simulink model "Calculator"  (R2024b)
settings: Solver=VariableStepAuto  StartTime=0.0  StopTime=10.0  RelTol=1e-3
(part 1 of 2)
settings Model: Creator=Ian  LastModifiedBy=Ian

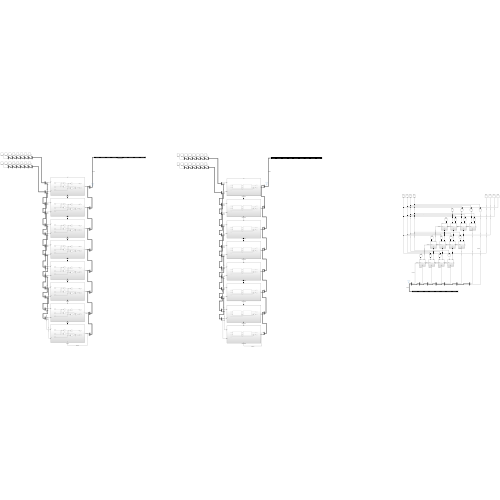
[thumbnail: Simulink's stored preview of the top-level diagram]
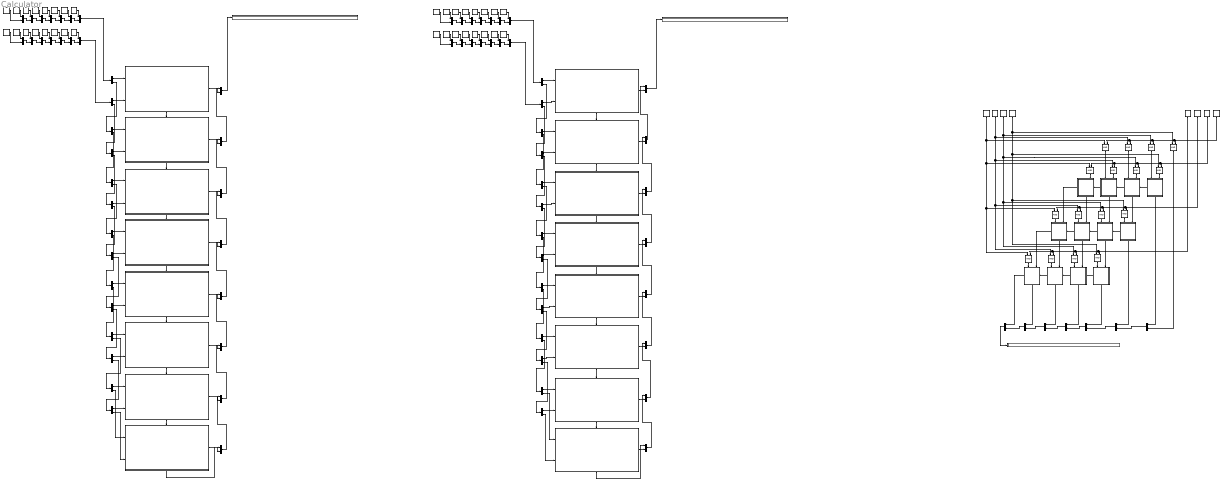
== system Calculator ==
  AND{,3..17} (16 alike) : Logic  IconShape=distinctive  AllPortsSameDT=off  OutDataTypeStr=boolean
  Add{11..13,15..18,21..25,27} (13 alike) : Constant  Value=0
  Add14 : Constant
  Add26 : Constant
  Add28 : Constant
  Adder : Subsystem
      settings: PortSchema="{\"entries\":[{\"content\":{\"sides\":[{\"content\":{\"connectorIds\":[\"In1\",\"In2\"]},\"type\":\"ConnectorPlacement.EquallySpacedRectSide\",\"uuid\":\"7bda4a13-5714-4766-b13e-fbedd8378c0d\"},{\"content\":{\"connectorIds\":[\"Out1\"],\"side\":\"RIGHT\"},\"type\":\"ConnectorPlacement.EquallySpacedRectSide\",\"uuid\":\"12590a9d-1e20-4d4b-a015-8cc67798c588\"},{\"content\":{\"connectorIds\":[\"In3\"],\"side\":\"TOP\"},\"type\":\"ConnectorPlacement.EquallySpacedRectSide\",\"uuid\":\"02eef574-06bf-4445-a216-f5494700e03c\"},{\"content\":{\"connectorIds\":[\"Out2\"],\"side\":\"BOTTOM\"},\"type\":\"ConnectorPlacement.EquallySpacedRectSide\",\"uuid\":\"95bb6c32-4776-4ae5-879f-000f498d11ec\"}]},\"type\":\"ConnectorPlacement.EquallySpacedConnector\",\"uuid\":\"b3982cbe-2d0c-455f-a3cf-748a4a59c66e\"}],\"packageUris\":[\"http://schema.mathworks.com/mf0/Connector/R2020b\"],\"version\":\"1.0\"}"
  Adder1 : Subsystem
      settings: PortSchema="{\"entries\":[{\"content\":{\"sides\":[{\"content\":{\"connectorIds\":[\"In1\",\"In2\"]},\"type\":\"ConnectorPlacement.EquallySpacedRectSide\",\"uuid\":\"7bda4a13-5714-4766-b13e-fbedd8378c0d\"},{\"content\":{\"connectorIds\":[\"Out1\"],\"side\":\"RIGHT\"},\"type\":\"ConnectorPlacement.EquallySpacedRectSide\",\"uuid\":\"12590a9d-1e20-4d4b-a015-8cc67798c588\"},{\"content\":{\"connectorIds\":[\"In3\"],\"side\":\"TOP\"},\"type\":\"ConnectorPlacement.EquallySpacedRectSide\",\"uuid\":\"02eef574-06bf-4445-a216-f5494700e03c\"},{\"content\":{\"connectorIds\":[\"Out2\"],\"side\":\"BOTTOM\"},\"type\":\"ConnectorPlacement.EquallySpacedRectSide\",\"uuid\":\"95bb6c32-4776-4ae5-879f-000f498d11ec\"}]},\"type\":\"ConnectorPlacement.EquallySpacedConnector\",\"uuid\":\"b3982cbe-2d0c-455f-a3cf-748a4a59c66e\"}],\"packageUris\":[\"http://schema.mathworks.com/mf0/Connector/R2020b\"],\"version\":\"1.0\"}"
  Adder10 : Subsystem
      settings: PortSchema="{\"entries\":[{\"content\":{\"sides\":[{\"content\":{\"connectorIds\":[\"In1\",\"In2\"]},\"type\":\"ConnectorPlacement.EquallySpacedRectSide\",\"uuid\":\"7bda4a13-5714-4766-b13e-fbedd8378c0d\"},{\"content\":{\"connectorIds\":[\"Out1\"],\"side\":\"RIGHT\"},\"type\":\"ConnectorPlacement.EquallySpacedRectSide\",\"uuid\":\"12590a9d-1e20-4d4b-a015-8cc67798c588\"},{\"content\":{\"connectorIds\":[\"In3\"],\"side\":\"TOP\"},\"type\":\"ConnectorPlacement.EquallySpacedRectSide\",\"uuid\":\"02eef574-06bf-4445-a216-f5494700e03c\"},{\"content\":{\"connectorIds\":[\"Out2\"],\"side\":\"BOTTOM\"},\"type\":\"ConnectorPlacement.EquallySpacedRectSide\",\"uuid\":\"95bb6c32-4776-4ae5-879f-000f498d11ec\"}]},\"type\":\"ConnectorPlacement.EquallySpacedConnector\",\"uuid\":\"b3982cbe-2d0c-455f-a3cf-748a4a59c66e\"}],\"packageUris\":[\"http://schema.mathworks.com/mf0/Connector/R2020b\"],\"version\":\"1.0\"}"
  Adder11 : Subsystem
      settings: PortSchema="{\"entries\":[{\"content\":{\"sides\":[{\"content\":{\"connectorIds\":[\"In1\",\"In2\"]},\"type\":\"ConnectorPlacement.EquallySpacedRectSide\",\"uuid\":\"7bda4a13-5714-4766-b13e-fbedd8378c0d\"},{\"content\":{\"connectorIds\":[\"Out1\"],\"side\":\"RIGHT\"},\"type\":\"ConnectorPlacement.EquallySpacedRectSide\",\"uuid\":\"12590a9d-1e20-4d4b-a015-8cc67798c588\"},{\"content\":{\"connectorIds\":[\"In3\"],\"side\":\"TOP\"},\"type\":\"ConnectorPlacement.EquallySpacedRectSide\",\"uuid\":\"02eef574-06bf-4445-a216-f5494700e03c\"},{\"content\":{\"connectorIds\":[\"Out2\"],\"side\":\"BOTTOM\"},\"type\":\"ConnectorPlacement.EquallySpacedRectSide\",\"uuid\":\"95bb6c32-4776-4ae5-879f-000f498d11ec\"}]},\"type\":\"ConnectorPlacement.EquallySpacedConnector\",\"uuid\":\"b3982cbe-2d0c-455f-a3cf-748a4a59c66e\"}],\"packageUris\":[\"http://schema.mathworks.com/mf0/Connector/R2020b\"],\"version\":\"1.0\"}"
  Adder12 : Subsystem
      settings: PortSchema="{\"entries\":[{\"content\":{\"sides\":[{\"content\":{\"connectorIds\":[\"In1\",\"In2\"]},\"type\":\"ConnectorPlacement.EquallySpacedRectSide\",\"uuid\":\"7bda4a13-5714-4766-b13e-fbedd8378c0d\"},{\"content\":{\"connectorIds\":[\"Out1\"],\"side\":\"RIGHT\"},\"type\":\"ConnectorPlacement.EquallySpacedRectSide\",\"uuid\":\"12590a9d-1e20-4d4b-a015-8cc67798c588\"},{\"content\":{\"connectorIds\":[\"In3\"],\"side\":\"TOP\"},\"type\":\"ConnectorPlacement.EquallySpacedRectSide\",\"uuid\":\"02eef574-06bf-4445-a216-f5494700e03c\"},{\"content\":{\"connectorIds\":[\"Out2\"],\"side\":\"BOTTOM\"},\"type\":\"ConnectorPlacement.EquallySpacedRectSide\",\"uuid\":\"95bb6c32-4776-4ae5-879f-000f498d11ec\"}]},\"type\":\"ConnectorPlacement.EquallySpacedConnector\",\"uuid\":\"b3982cbe-2d0c-455f-a3cf-748a4a59c66e\"}],\"packageUris\":[\"http://schema.mathworks.com/mf0/Connector/R2020b\"],\"version\":\"1.0\"}"
  Adder13 : Subsystem
      settings: PortSchema="{\"entries\":[{\"content\":{\"sides\":[{\"content\":{\"connectorIds\":[\"In1\",\"In2\"]},\"type\":\"ConnectorPlacement.EquallySpacedRectSide\",\"uuid\":\"7bda4a13-5714-4766-b13e-fbedd8378c0d\"},{\"content\":{\"connectorIds\":[\"Out1\"],\"side\":\"RIGHT\"},\"type\":\"ConnectorPlacement.EquallySpacedRectSide\",\"uuid\":\"12590a9d-1e20-4d4b-a015-8cc67798c588\"},{\"content\":{\"connectorIds\":[\"In3\"],\"side\":\"TOP\"},\"type\":\"ConnectorPlacement.EquallySpacedRectSide\",\"uuid\":\"02eef574-06bf-4445-a216-f5494700e03c\"},{\"content\":{\"connectorIds\":[\"Out2\"],\"side\":\"BOTTOM\"},\"type\":\"ConnectorPlacement.EquallySpacedRectSide\",\"uuid\":\"95bb6c32-4776-4ae5-879f-000f498d11ec\"}]},\"type\":\"ConnectorPlacement.EquallySpacedConnector\",\"uuid\":\"b3982cbe-2d0c-455f-a3cf-748a4a59c66e\"}],\"packageUris\":[\"http://schema.mathworks.com/mf0/Connector/R2020b\"],\"version\":\"1.0\"}"
  Adder14 : Subsystem
      settings: PortSchema="{\"entries\":[{\"content\":{\"sides\":[{\"content\":{\"connectorIds\":[\"In1\",\"In2\"]},\"type\":\"ConnectorPlacement.EquallySpacedRectSide\",\"uuid\":\"7bda4a13-5714-4766-b13e-fbedd8378c0d\"},{\"content\":{\"connectorIds\":[\"Out1\"],\"side\":\"RIGHT\"},\"type\":\"ConnectorPlacement.EquallySpacedRectSide\",\"uuid\":\"12590a9d-1e20-4d4b-a015-8cc67798c588\"},{\"content\":{\"connectorIds\":[\"In3\"],\"side\":\"TOP\"},\"type\":\"ConnectorPlacement.EquallySpacedRectSide\",\"uuid\":\"02eef574-06bf-4445-a216-f5494700e03c\"},{\"content\":{\"connectorIds\":[\"Out2\"],\"side\":\"BOTTOM\"},\"type\":\"ConnectorPlacement.EquallySpacedRectSide\",\"uuid\":\"95bb6c32-4776-4ae5-879f-000f498d11ec\"}]},\"type\":\"ConnectorPlacement.EquallySpacedConnector\",\"uuid\":\"b3982cbe-2d0c-455f-a3cf-748a4a59c66e\"}],\"packageUris\":[\"http://schema.mathworks.com/mf0/Connector/R2020b\"],\"version\":\"1.0\"}"
  Adder15 : Subsystem
      settings: PortSchema="{\"entries\":[{\"content\":{\"sides\":[{\"content\":{\"connectorIds\":[\"In1\",\"In2\"]},\"type\":\"ConnectorPlacement.EquallySpacedRectSide\",\"uuid\":\"7bda4a13-5714-4766-b13e-fbedd8378c0d\"},{\"content\":{\"connectorIds\":[\"Out1\"],\"side\":\"RIGHT\"},\"type\":\"ConnectorPlacement.EquallySpacedRectSide\",\"uuid\":\"12590a9d-1e20-4d4b-a015-8cc67798c588\"},{\"content\":{\"connectorIds\":[\"In3\"],\"side\":\"TOP\"},\"type\":\"ConnectorPlacement.EquallySpacedRectSide\",\"uuid\":\"02eef574-06bf-4445-a216-f5494700e03c\"},{\"content\":{\"connectorIds\":[\"Out2\"],\"side\":\"BOTTOM\"},\"type\":\"ConnectorPlacement.EquallySpacedRectSide\",\"uuid\":\"95bb6c32-4776-4ae5-879f-000f498d11ec\"}]},\"type\":\"ConnectorPlacement.EquallySpacedConnector\",\"uuid\":\"b3982cbe-2d0c-455f-a3cf-748a4a59c66e\"}],\"packageUris\":[\"http://schema.mathworks.com/mf0/Connector/R2020b\"],\"version\":\"1.0\"}"
  Adder16 : Subsystem
      settings: PortSchema="{\"entries\":[{\"content\":{\"sides\":[{\"content\":{\"connectorIds\":[\"In1\",\"In2\"]},\"type\":\"ConnectorPlacement.EquallySpacedRectSide\",\"uuid\":\"7bda4a13-5714-4766-b13e-fbedd8378c0d\"},{\"content\":{\"connectorIds\":[\"Out1\"],\"side\":\"RIGHT\"},\"type\":\"ConnectorPlacement.EquallySpacedRectSide\",\"uuid\":\"12590a9d-1e20-4d4b-a015-8cc67798c588\"},{\"content\":{\"connectorIds\":[\"In3\"],\"side\":\"TOP\"},\"type\":\"ConnectorPlacement.EquallySpacedRectSide\",\"uuid\":\"02eef574-06bf-4445-a216-f5494700e03c\"},{\"content\":{\"connectorIds\":[\"Out2\"],\"side\":\"BOTTOM\"},\"type\":\"ConnectorPlacement.EquallySpacedRectSide\",\"uuid\":\"95bb6c32-4776-4ae5-879f-000f498d11ec\"}]},\"type\":\"ConnectorPlacement.EquallySpacedConnector\",\"uuid\":\"b3982cbe-2d0c-455f-a3cf-748a4a59c66e\"}],\"packageUris\":[\"http://schema.mathworks.com/mf0/Connector/R2020b\"],\"version\":\"1.0\"}"
  Adder17 : Subsystem
      settings: PortSchema="{\"entries\":[{\"content\":{\"sides\":[{\"content\":{\"connectorIds\":[\"In1\",\"In2\"]},\"type\":\"ConnectorPlacement.EquallySpacedRectSide\",\"uuid\":\"7bda4a13-5714-4766-b13e-fbedd8378c0d\"},{\"content\":{\"connectorIds\":[\"Out1\"],\"side\":\"RIGHT\"},\"type\":\"ConnectorPlacement.EquallySpacedRectSide\",\"uuid\":\"12590a9d-1e20-4d4b-a015-8cc67798c588\"},{\"content\":{\"connectorIds\":[\"In3\"],\"side\":\"TOP\"},\"type\":\"ConnectorPlacement.EquallySpacedRectSide\",\"uuid\":\"02eef574-06bf-4445-a216-f5494700e03c\"},{\"content\":{\"connectorIds\":[\"Out2\"],\"side\":\"BOTTOM\"},\"type\":\"ConnectorPlacement.EquallySpacedRectSide\",\"uuid\":\"95bb6c32-4776-4ae5-879f-000f498d11ec\"}]},\"type\":\"ConnectorPlacement.EquallySpacedConnector\",\"uuid\":\"b3982cbe-2d0c-455f-a3cf-748a4a59c66e\"}],\"packageUris\":[\"http://schema.mathworks.com/mf0/Connector/R2020b\"],\"version\":\"1.0\"}"
  Adder18 : Subsystem
      settings: PortSchema="{\"entries\":[{\"content\":{\"sides\":[{\"content\":{\"connectorIds\":[\"In1\",\"In2\"]},\"type\":\"ConnectorPlacement.EquallySpacedRectSide\",\"uuid\":\"7bda4a13-5714-4766-b13e-fbedd8378c0d\"},{\"content\":{\"connectorIds\":[\"Out1\"],\"side\":\"RIGHT\"},\"type\":\"ConnectorPlacement.EquallySpacedRectSide\",\"uuid\":\"12590a9d-1e20-4d4b-a015-8cc67798c588\"},{\"content\":{\"connectorIds\":[\"In3\"],\"side\":\"TOP\"},\"type\":\"ConnectorPlacement.EquallySpacedRectSide\",\"uuid\":\"02eef574-06bf-4445-a216-f5494700e03c\"},{\"content\":{\"connectorIds\":[\"Out2\"],\"side\":\"BOTTOM\"},\"type\":\"ConnectorPlacement.EquallySpacedRectSide\",\"uuid\":\"95bb6c32-4776-4ae5-879f-000f498d11ec\"}]},\"type\":\"ConnectorPlacement.EquallySpacedConnector\",\"uuid\":\"b3982cbe-2d0c-455f-a3cf-748a4a59c66e\"}],\"packageUris\":[\"http://schema.mathworks.com/mf0/Connector/R2020b\"],\"version\":\"1.0\"}"
  Adder19 : Subsystem
      settings: PortSchema="{\"entries\":[{\"content\":{\"sides\":[{\"content\":{\"connectorIds\":[\"In1\",\"In2\"]},\"type\":\"ConnectorPlacement.EquallySpacedRectSide\",\"uuid\":\"7bda4a13-5714-4766-b13e-fbedd8378c0d\"},{\"content\":{\"connectorIds\":[\"Out1\"],\"side\":\"RIGHT\"},\"type\":\"ConnectorPlacement.EquallySpacedRectSide\",\"uuid\":\"12590a9d-1e20-4d4b-a015-8cc67798c588\"},{\"content\":{\"connectorIds\":[\"In3\"],\"side\":\"TOP\"},\"type\":\"ConnectorPlacement.EquallySpacedRectSide\",\"uuid\":\"02eef574-06bf-4445-a216-f5494700e03c\"},{\"content\":{\"connectorIds\":[\"Out2\"],\"side\":\"BOTTOM\"},\"type\":\"ConnectorPlacement.EquallySpacedRectSide\",\"uuid\":\"95bb6c32-4776-4ae5-879f-000f498d11ec\"}]},\"type\":\"ConnectorPlacement.EquallySpacedConnector\",\"uuid\":\"b3982cbe-2d0c-455f-a3cf-748a4a59c66e\"}],\"packageUris\":[\"http://schema.mathworks.com/mf0/Connector/R2020b\"],\"version\":\"1.0\"}"
  Adder2 : Subsystem
      settings: PortSchema="{\"entries\":[{\"content\":{\"sides\":[{\"content\":{\"connectorIds\":[\"In1\",\"In2\"]},\"type\":\"ConnectorPlacement.EquallySpacedRectSide\",\"uuid\":\"7bda4a13-5714-4766-b13e-fbedd8378c0d\"},{\"content\":{\"connectorIds\":[\"Out1\"],\"side\":\"RIGHT\"},\"type\":\"ConnectorPlacement.EquallySpacedRectSide\",\"uuid\":\"12590a9d-1e20-4d4b-a015-8cc67798c588\"},{\"content\":{\"connectorIds\":[\"In3\"],\"side\":\"TOP\"},\"type\":\"ConnectorPlacement.EquallySpacedRectSide\",\"uuid\":\"02eef574-06bf-4445-a216-f5494700e03c\"},{\"content\":{\"connectorIds\":[\"Out2\"],\"side\":\"BOTTOM\"},\"type\":\"ConnectorPlacement.EquallySpacedRectSide\",\"uuid\":\"95bb6c32-4776-4ae5-879f-000f498d11ec\"}]},\"type\":\"ConnectorPlacement.EquallySpacedConnector\",\"uuid\":\"b3982cbe-2d0c-455f-a3cf-748a4a59c66e\"}],\"packageUris\":[\"http://schema.mathworks.com/mf0/Connector/R2020b\"],\"version\":\"1.0\"}"
  Adder3 : Subsystem
      settings: PortSchema="{\"entries\":[{\"content\":{\"sides\":[{\"content\":{\"connectorIds\":[\"In1\",\"In2\"]},\"type\":\"ConnectorPlacement.EquallySpacedRectSide\",\"uuid\":\"7bda4a13-5714-4766-b13e-fbedd8378c0d\"},{\"content\":{\"connectorIds\":[\"Out1\"],\"side\":\"RIGHT\"},\"type\":\"ConnectorPlacement.EquallySpacedRectSide\",\"uuid\":\"12590a9d-1e20-4d4b-a015-8cc67798c588\"},{\"content\":{\"connectorIds\":[\"In3\"],\"side\":\"TOP\"},\"type\":\"ConnectorPlacement.EquallySpacedRectSide\",\"uuid\":\"02eef574-06bf-4445-a216-f5494700e03c\"},{\"content\":{\"connectorIds\":[\"Out2\"],\"side\":\"BOTTOM\"},\"type\":\"ConnectorPlacement.EquallySpacedRectSide\",\"uuid\":\"95bb6c32-4776-4ae5-879f-000f498d11ec\"}]},\"type\":\"ConnectorPlacement.EquallySpacedConnector\",\"uuid\":\"b3982cbe-2d0c-455f-a3cf-748a4a59c66e\"}],\"packageUris\":[\"http://schema.mathworks.com/mf0/Connector/R2020b\"],\"version\":\"1.0\"}"
  Adder4 : Subsystem
      settings: PortSchema="{\"entries\":[{\"content\":{\"sides\":[{\"content\":{\"connectorIds\":[\"In1\",\"In2\"]},\"type\":\"ConnectorPlacement.EquallySpacedRectSide\",\"uuid\":\"7bda4a13-5714-4766-b13e-fbedd8378c0d\"},{\"content\":{\"connectorIds\":[\"Out1\"],\"side\":\"RIGHT\"},\"type\":\"ConnectorPlacement.EquallySpacedRectSide\",\"uuid\":\"12590a9d-1e20-4d4b-a015-8cc67798c588\"},{\"content\":{\"connectorIds\":[\"In3\"],\"side\":\"TOP\"},\"type\":\"ConnectorPlacement.EquallySpacedRectSide\",\"uuid\":\"02eef574-06bf-4445-a216-f5494700e03c\"},{\"content\":{\"connectorIds\":[\"Out2\"],\"side\":\"BOTTOM\"},\"type\":\"ConnectorPlacement.EquallySpacedRectSide\",\"uuid\":\"95bb6c32-4776-4ae5-879f-000f498d11ec\"}]},\"type\":\"ConnectorPlacement.EquallySpacedConnector\",\"uuid\":\"b3982cbe-2d0c-455f-a3cf-748a4a59c66e\"}],\"packageUris\":[\"http://schema.mathworks.com/mf0/Connector/R2020b\"],\"version\":\"1.0\"}"
  Adder5 : Subsystem
      settings: PortSchema="{\"entries\":[{\"content\":{\"sides\":[{\"content\":{\"connectorIds\":[\"In1\",\"In2\"]},\"type\":\"ConnectorPlacement.EquallySpacedRectSide\",\"uuid\":\"7bda4a13-5714-4766-b13e-fbedd8378c0d\"},{\"content\":{\"connectorIds\":[\"Out1\"],\"side\":\"RIGHT\"},\"type\":\"ConnectorPlacement.EquallySpacedRectSide\",\"uuid\":\"12590a9d-1e20-4d4b-a015-8cc67798c588\"},{\"content\":{\"connectorIds\":[\"In3\"],\"side\":\"TOP\"},\"type\":\"ConnectorPlacement.EquallySpacedRectSide\",\"uuid\":\"02eef574-06bf-4445-a216-f5494700e03c\"},{\"content\":{\"connectorIds\":[\"Out2\"],\"side\":\"BOTTOM\"},\"type\":\"ConnectorPlacement.EquallySpacedRectSide\",\"uuid\":\"95bb6c32-4776-4ae5-879f-000f498d11ec\"}]},\"type\":\"ConnectorPlacement.EquallySpacedConnector\",\"uuid\":\"b3982cbe-2d0c-455f-a3cf-748a4a59c66e\"}],\"packageUris\":[\"http://schema.mathworks.com/mf0/Connector/R2020b\"],\"version\":\"1.0\"}"
  Adder6 : Subsystem
      settings: PortSchema="{\"entries\":[{\"content\":{\"sides\":[{\"content\":{\"connectorIds\":[\"In1\",\"In2\"]},\"type\":\"ConnectorPlacement.EquallySpacedRectSide\",\"uuid\":\"7bda4a13-5714-4766-b13e-fbedd8378c0d\"},{\"content\":{\"connectorIds\":[\"Out1\"],\"side\":\"RIGHT\"},\"type\":\"ConnectorPlacement.EquallySpacedRectSide\",\"uuid\":\"12590a9d-1e20-4d4b-a015-8cc67798c588\"},{\"content\":{\"connectorIds\":[\"In3\"],\"side\":\"TOP\"},\"type\":\"ConnectorPlacement.EquallySpacedRectSide\",\"uuid\":\"02eef574-06bf-4445-a216-f5494700e03c\"},{\"content\":{\"connectorIds\":[\"Out2\"],\"side\":\"BOTTOM\"},\"type\":\"ConnectorPlacement.EquallySpacedRectSide\",\"uuid\":\"95bb6c32-4776-4ae5-879f-000f498d11ec\"}]},\"type\":\"ConnectorPlacement.EquallySpacedConnector\",\"uuid\":\"b3982cbe-2d0c-455f-a3cf-748a4a59c66e\"}],\"packageUris\":[\"http://schema.mathworks.com/mf0/Connector/R2020b\"],\"version\":\"1.0\"}"
  Adder7 : Subsystem
      settings: PortSchema="{\"entries\":[{\"content\":{\"sides\":[{\"content\":{\"connectorIds\":[\"In1\",\"In2\"]},\"type\":\"ConnectorPlacement.EquallySpacedRectSide\",\"uuid\":\"7bda4a13-5714-4766-b13e-fbedd8378c0d\"},{\"content\":{\"connectorIds\":[\"Out1\"],\"side\":\"RIGHT\"},\"type\":\"ConnectorPlacement.EquallySpacedRectSide\",\"uuid\":\"12590a9d-1e20-4d4b-a015-8cc67798c588\"},{\"content\":{\"connectorIds\":[\"In3\"],\"side\":\"TOP\"},\"type\":\"ConnectorPlacement.EquallySpacedRectSide\",\"uuid\":\"02eef574-06bf-4445-a216-f5494700e03c\"},{\"content\":{\"connectorIds\":[\"Out2\"],\"side\":\"BOTTOM\"},\"type\":\"ConnectorPlacement.EquallySpacedRectSide\",\"uuid\":\"95bb6c32-4776-4ae5-879f-000f498d11ec\"}]},\"type\":\"ConnectorPlacement.EquallySpacedConnector\",\"uuid\":\"b3982cbe-2d0c-455f-a3cf-748a4a59c66e\"}],\"packageUris\":[\"http://schema.mathworks.com/mf0/Connector/R2020b\"],\"version\":\"1.0\"}"
  Adder8 : Subsystem
      settings: PortSchema="{\"entries\":[{\"content\":{\"sides\":[{\"content\":{\"connectorIds\":[\"In1\",\"In2\"]},\"type\":\"ConnectorPlacement.EquallySpacedRectSide\",\"uuid\":\"7bda4a13-5714-4766-b13e-fbedd8378c0d\"},{\"content\":{\"connectorIds\":[\"Out1\"],\"side\":\"RIGHT\"},\"type\":\"ConnectorPlacement.EquallySpacedRectSide\",\"uuid\":\"12590a9d-1e20-4d4b-a015-8cc67798c588\"},{\"content\":{\"connectorIds\":[\"In3\"],\"side\":\"TOP\"},\"type\":\"ConnectorPlacement.EquallySpacedRectSide\",\"uuid\":\"02eef574-06bf-4445-a216-f5494700e03c\"},{\"content\":{\"connectorIds\":[\"Out2\"],\"side\":\"BOTTOM\"},\"type\":\"ConnectorPlacement.EquallySpacedRectSide\",\"uuid\":\"95bb6c32-4776-4ae5-879f-000f498d11ec\"}]},\"type\":\"ConnectorPlacement.EquallySpacedConnector\",\"uuid\":\"b3982cbe-2d0c-455f-a3cf-748a4a59c66e\"}],\"packageUris\":[\"http://schema.mathworks.com/mf0/Connector/R2020b\"],\"version\":\"1.0\"}"
  Adder9 : Subsystem
      settings: PortSchema="{\"entries\":[{\"content\":{\"sides\":[{\"content\":{\"connectorIds\":[\"In1\",\"In2\"]},\"type\":\"ConnectorPlacement.EquallySpacedRectSide\",\"uuid\":\"7bda4a13-5714-4766-b13e-fbedd8378c0d\"},{\"content\":{\"connectorIds\":[\"Out1\"],\"side\":\"RIGHT\"},\"type\":\"ConnectorPlacement.EquallySpacedRectSide\",\"uuid\":\"12590a9d-1e20-4d4b-a015-8cc67798c588\"},{\"content\":{\"connectorIds\":[\"In3\"],\"side\":\"TOP\"},\"type\":\"ConnectorPlacement.EquallySpacedRectSide\",\"uuid\":\"02eef574-06bf-4445-a216-f5494700e03c\"},{\"content\":{\"connectorIds\":[\"Out2\"],\"side\":\"BOTTOM\"},\"type\":\"ConnectorPlacement.EquallySpacedRectSide\",\"uuid\":\"95bb6c32-4776-4ae5-879f-000f498d11ec\"}]},\"type\":\"ConnectorPlacement.EquallySpacedConnector\",\"uuid\":\"b3982cbe-2d0c-455f-a3cf-748a4a59c66e\"}],\"packageUris\":[\"http://schema.mathworks.com/mf0/Connector/R2020b\"],\"version\":\"1.0\"}"
  AdditionDisplay : Display
  Bus Creator{,1..50} (51 alike) : BusCreator  Inputs=2
  Bus Selector{,1..27} (28 alike) : BusSelector  OutputSignals=signal1,signal2
  Display : Display
  Display1 : Display
  Mult{11..14,24} (5 alike) : Constant
  Mult21 : Constant  Value=0
  Mult22 : Constant  Value=0
  Mult23 : Constant  Value=0
  Sub{11..14,16,18,21..24,26,28} (12 alike) : Constant  Value=0
  Sub{15,17,25,27} (4 alike) : Constant
  Subtractor1 : Subsystem
      settings: PortSchema="{\"entries\":[{\"content\":{\"sides\":[{\"content\":{\"connectorIds\":[\"In1\",\"In2\"]},\"type\":\"ConnectorPlacement.EquallySpacedRectSide\",\"uuid\":\"7bda4a13-5714-4766-b13e-fbedd8378c0d\"},{\"content\":{\"connectorIds\":[\"Out1\"],\"side\":\"RIGHT\"},\"type\":\"ConnectorPlacement.EquallySpacedRectSide\",\"uuid\":\"12590a9d-1e20-4d4b-a015-8cc67798c588\"},{\"content\":{\"connectorIds\":[\"In3\"],\"side\":\"TOP\"},\"type\":\"ConnectorPlacement.EquallySpacedRectSide\",\"uuid\":\"02eef574-06bf-4445-a216-f5494700e03c\"},{\"content\":{\"connectorIds\":[\"Out2\"],\"side\":\"BOTTOM\"},\"type\":\"ConnectorPlacement.EquallySpacedRectSide\",\"uuid\":\"e8f31c1b-a942-47d5-ae1c-1de8906fe25d\"}]},\"type\":\"ConnectorPlacement.EquallySpacedConnector\",\"uuid\":\"b3982cbe-2d0c-455f-a3cf-748a4a59c66e\"}],\"packageUris\":[\"http://schema.mathworks.com/mf0/Connector/R2020b\"],\"version\":\"1.0\"}"
  Subtractor2 : Subsystem
      settings: PortSchema="{\"entries\":[{\"content\":{\"sides\":[{\"content\":{\"connectorIds\":[\"In1\",\"In2\"]},\"type\":\"ConnectorPlacement.EquallySpacedRectSide\",\"uuid\":\"7bda4a13-5714-4766-b13e-fbedd8378c0d\"},{\"content\":{\"connectorIds\":[\"Out1\"],\"side\":\"RIGHT\"},\"type\":\"ConnectorPlacement.EquallySpacedRectSide\",\"uuid\":\"12590a9d-1e20-4d4b-a015-8cc67798c588\"},{\"content\":{\"connectorIds\":[\"In3\"],\"side\":\"TOP\"},\"type\":\"ConnectorPlacement.EquallySpacedRectSide\",\"uuid\":\"02eef574-06bf-4445-a216-f5494700e03c\"},{\"content\":{\"connectorIds\":[\"Out2\"],\"side\":\"BOTTOM\"},\"type\":\"ConnectorPlacement.EquallySpacedRectSide\",\"uuid\":\"e8f31c1b-a942-47d5-ae1c-1de8906fe25d\"}]},\"type\":\"ConnectorPlacement.EquallySpacedConnector\",\"uuid\":\"b3982cbe-2d0c-455f-a3cf-748a4a59c66e\"}],\"packageUris\":[\"http://schema.mathworks.com/mf0/Connector/R2020b\"],\"version\":\"1.0\"}"
  Subtractor3 : Subsystem
      settings: PortSchema="{\"entries\":[{\"content\":{\"sides\":[{\"content\":{\"connectorIds\":[\"In1\",\"In2\"]},\"type\":\"ConnectorPlacement.EquallySpacedRectSide\",\"uuid\":\"7bda4a13-5714-4766-b13e-fbedd8378c0d\"},{\"content\":{\"connectorIds\":[\"Out1\"],\"side\":\"RIGHT\"},\"type\":\"ConnectorPlacement.EquallySpacedRectSide\",\"uuid\":\"12590a9d-1e20-4d4b-a015-8cc67798c588\"},{\"content\":{\"connectorIds\":[\"In3\"],\"side\":\"TOP\"},\"type\":\"ConnectorPlacement.EquallySpacedRectSide\",\"uuid\":\"02eef574-06bf-4445-a216-f5494700e03c\"},{\"content\":{\"connectorIds\":[\"Out2\"],\"side\":\"BOTTOM\"},\"type\":\"ConnectorPlacement.EquallySpacedRectSide\",\"uuid\":\"e8f31c1b-a942-47d5-ae1c-1de8906fe25d\"}]},\"type\":\"ConnectorPlacement.EquallySpacedConnector\",\"uuid\":\"b3982cbe-2d0c-455f-a3cf-748a4a59c66e\"}],\"packageUris\":[\"http://schema.mathworks.com/mf0/Connector/R2020b\"],\"version\":\"1.0\"}"
  Subtractor4 : Subsystem
      settings: PortSchema="{\"entries\":[{\"content\":{\"sides\":[{\"content\":{\"connectorIds\":[\"In1\",\"In2\"]},\"type\":\"ConnectorPlacement.EquallySpacedRectSide\",\"uuid\":\"7bda4a13-5714-4766-b13e-fbedd8378c0d\"},{\"content\":{\"connectorIds\":[\"Out1\"],\"side\":\"RIGHT\"},\"type\":\"ConnectorPlacement.EquallySpacedRectSide\",\"uuid\":\"12590a9d-1e20-4d4b-a015-8cc67798c588\"},{\"content\":{\"connectorIds\":[\"In3\"],\"side\":\"TOP\"},\"type\":\"ConnectorPlacement.EquallySpacedRectSide\",\"uuid\":\"02eef574-06bf-4445-a216-f5494700e03c\"},{\"content\":{\"connectorIds\":[\"Out2\"],\"side\":\"BOTTOM\"},\"type\":\"ConnectorPlacement.EquallySpacedRectSide\",\"uuid\":\"e8f31c1b-a942-47d5-ae1c-1de8906fe25d\"}]},\"type\":\"ConnectorPlacement.EquallySpacedConnector\",\"uuid\":\"b3982cbe-2d0c-455f-a3cf-748a4a59c66e\"}],\"packageUris\":[\"http://schema.mathworks.com/mf0/Connector/R2020b\"],\"version\":\"1.0\"}"
  Subtractor5 : Subsystem
      settings: PortSchema="{\"entries\":[{\"content\":{\"sides\":[{\"content\":{\"connectorIds\":[\"In1\",\"In2\"]},\"type\":\"ConnectorPlacement.EquallySpacedRectSide\",\"uuid\":\"7bda4a13-5714-4766-b13e-fbedd8378c0d\"},{\"content\":{\"connectorIds\":[\"Out1\"],\"side\":\"RIGHT\"},\"type\":\"ConnectorPlacement.EquallySpacedRectSide\",\"uuid\":\"12590a9d-1e20-4d4b-a015-8cc67798c588\"},{\"content\":{\"connectorIds\":[\"In3\"],\"side\":\"TOP\"},\"type\":\"ConnectorPlacement.EquallySpacedRectSide\",\"uuid\":\"02eef574-06bf-4445-a216-f5494700e03c\"},{\"content\":{\"connectorIds\":[\"Out2\"],\"side\":\"BOTTOM\"},\"type\":\"ConnectorPlacement.EquallySpacedRectSide\",\"uuid\":\"e8f31c1b-a942-47d5-ae1c-1de8906fe25d\"}]},\"type\":\"ConnectorPlacement.EquallySpacedConnector\",\"uuid\":\"b3982cbe-2d0c-455f-a3cf-748a4a59c66e\"}],\"packageUris\":[\"http://schema.mathworks.com/mf0/Connector/R2020b\"],\"version\":\"1.0\"}"
  Subtractor6 : Subsystem
      settings: PortSchema="{\"entries\":[{\"content\":{\"sides\":[{\"content\":{\"connectorIds\":[\"In1\",\"In2\"]},\"type\":\"ConnectorPlacement.EquallySpacedRectSide\",\"uuid\":\"7bda4a13-5714-4766-b13e-fbedd8378c0d\"},{\"content\":{\"connectorIds\":[\"Out1\"],\"side\":\"RIGHT\"},\"type\":\"ConnectorPlacement.EquallySpacedRectSide\",\"uuid\":\"12590a9d-1e20-4d4b-a015-8cc67798c588\"},{\"content\":{\"connectorIds\":[\"In3\"],\"side\":\"TOP\"},\"type\":\"ConnectorPlacement.EquallySpacedRectSide\",\"uuid\":\"02eef574-06bf-4445-a216-f5494700e03c\"},{\"content\":{\"connectorIds\":[\"Out2\"],\"side\":\"BOTTOM\"},\"type\":\"ConnectorPlacement.EquallySpacedRectSide\",\"uuid\":\"e8f31c1b-a942-47d5-ae1c-1de8906fe25d\"}]},\"type\":\"ConnectorPlacement.EquallySpacedConnector\",\"uuid\":\"b3982cbe-2d0c-455f-a3cf-748a4a59c66e\"}],\"packageUris\":[\"http://schema.mathworks.com/mf0/Connector/R2020b\"],\"version\":\"1.0\"}"
  Subtractor7 : Subsystem
      settings: PortSchema="{\"entries\":[{\"content\":{\"sides\":[{\"content\":{\"connectorIds\":[\"In1\",\"In2\"]},\"type\":\"ConnectorPlacement.EquallySpacedRectSide\",\"uuid\":\"7bda4a13-5714-4766-b13e-fbedd8378c0d\"},{\"content\":{\"connectorIds\":[\"Out1\"],\"side\":\"RIGHT\"},\"type\":\"ConnectorPlacement.EquallySpacedRectSide\",\"uuid\":\"12590a9d-1e20-4d4b-a015-8cc67798c588\"},{\"content\":{\"connectorIds\":[\"In3\"],\"side\":\"TOP\"},\"type\":\"ConnectorPlacement.EquallySpacedRectSide\",\"uuid\":\"02eef574-06bf-4445-a216-f5494700e03c\"},{\"content\":{\"connectorIds\":[\"Out2\"],\"side\":\"BOTTOM\"},\"type\":\"ConnectorPlacement.EquallySpacedRectSide\",\"uuid\":\"e8f31c1b-a942-47d5-ae1c-1de8906fe25d\"}]},\"type\":\"ConnectorPlacement.EquallySpacedConnector\",\"uuid\":\"b3982cbe-2d0c-455f-a3cf-748a4a59c66e\"}],\"packageUris\":[\"http://schema.mathworks.com/mf0/Connector/R2020b\"],\"version\":\"1.0\"}"
  Subtractor8 : Subsystem
      settings: PortSchema="{\"entries\":[{\"content\":{\"sides\":[{\"content\":{\"connectorIds\":[\"In1\",\"In2\"]},\"type\":\"ConnectorPlacement.EquallySpacedRectSide\",\"uuid\":\"7bda4a13-5714-4766-b13e-fbedd8378c0d\"},{\"content\":{\"connectorIds\":[\"Out1\"],\"side\":\"RIGHT\"},\"type\":\"ConnectorPlacement.EquallySpacedRectSide\",\"uuid\":\"12590a9d-1e20-4d4b-a015-8cc67798c588\"},{\"content\":{\"connectorIds\":[\"In3\"],\"side\":\"TOP\"},\"type\":\"ConnectorPlacement.EquallySpacedRectSide\",\"uuid\":\"02eef574-06bf-4445-a216-f5494700e03c\"},{\"content\":{\"connectorIds\":[\"Out2\"],\"side\":\"BOTTOM\"},\"type\":\"ConnectorPlacement.EquallySpacedRectSide\",\"uuid\":\"e8f31c1b-a942-47d5-ae1c-1de8906fe25d\"}]},\"type\":\"ConnectorPlacement.EquallySpacedConnector\",\"uuid\":\"b3982cbe-2d0c-455f-a3cf-748a4a59c66e\"}],\"packageUris\":[\"http://schema.mathworks.com/mf0/Connector/R2020b\"],\"version\":\"1.0\"}"
  wires:
  Adder/2(Out2) -> Adder1/3(In3)
  Adder1/2(Out2) -> Adder2/3(In3)
  Adder2/2(Out2) -> Adder3/3(In3)
  Adder5/2(Out2) -> Adder6/3(In3)
  Adder6/2(Out2) -> Adder7/3(In3)
  Adder4/2(Out2) -> Adder5/3(In3)
  Adder3/2(Out2) -> Adder4/3(In3)
  Add12/1 -> Bus Creator8/1
  Add11/1 -> Bus Creator8/2
  Add13/1 -> Bus Creator9/1
  Bus Creator8/1 -> Bus Creator9/2
  Add15/1 -> Bus Creator11/1
  Add14/1 -> Bus Creator10/1
  Bus Creator9/1 -> Bus Creator10/2
  Bus Creator10/1 -> Bus Creator11/2
  Add16/1 -> Bus Creator14/1
  Add17/1 -> Bus Creator12/1
  Add18/1 -> Bus Creator13/1
  Bus Creator11/1 -> Bus Creator14/2
  Bus Creator14/1 -> Bus Creator12/2
  Bus Creator12/1 -> Bus Creator13/2
  Bus Creator19/1 -> Bus Creator17/2
  Bus Creator17/1 -> Bus Creator18/2
  Add23/1 -> Bus Creator21/1
  Add28/1 -> Bus Creator18/1
  Bus Creator20/1 -> Bus Creator21/2
  Bus Creator16/1 -> Bus Creator19/2
  Add25/1 -> Bus Creator16/1
  Add27/1 -> Bus Creator17/1
  Bus Creator21/1 -> Bus Creator15/2
  Add24/1 -> Bus Creator15/1
  Add22/1 -> Bus Creator20/1
  Add21/1 -> Bus Creator20/2
  Bus Creator15/1 -> Bus Creator16/2
  Add26/1 -> Bus Creator19/1
  Bus Selector/1 -> Adder/1(In1)  "<signal1>"
  Bus Selector/2 -> Bus Selector1/1  "<signal2>"
  Bus Selector2/1 -> Adder/2(In2)  "<signal1>"
  Bus Selector2/2 -> Bus Selector3/1  "<signal2>"
  Bus Selector1/1 -> Adder1/1(In1)  "<signal1>"
  Bus Selector3/1 -> Adder1/2(In2)  "<signal1>"
  Bus Selector6/2 -> Bus Selector7/1  "<signal2>"
  Bus Selector5/1 -> Adder3/1(In1)  "<signal1>"
  Bus Selector7/1 -> Adder3/2(In2)  "<signal1>"
  Bus Selector4/1 -> Adder2/1(In1)  "<signal1>"
  Bus Selector4/2 -> Bus Selector5/1  "<signal2>"
  Bus Selector6/1 -> Adder2/2(In2)  "<signal1>"
  Bus Selector3/2 -> Bus Selector6/1  "<signal2>"
  Bus Selector1/2 -> Bus Selector4/1  "<signal2>"
  Bus Selector8/2 -> Bus Selector10/1  "<signal2>"
  Bus Selector9/2 -> Bus Selector12/1  "<signal2>"
  Bus Selector10/2 -> Bus Selector11/1  "<signal2>"
  Bus Selector12/2 -> Bus Selector13/1  "<signal2>"
  Bus Selector5/2 -> Bus Selector8/1  "<signal2>"
  Bus Selector7/2 -> Bus Selector9/1  "<signal2>"
  Bus Selector8/1 -> Adder4/1(In1)  "<signal1>"
  Bus Selector9/1 -> Adder4/2(In2)  "<signal1>"
  Bus Selector13/1 -> Adder6/2(In2)  "<signal1>"
  Bus Selector11/1 -> Adder6/1(In1)  "<signal1>"
  Bus Selector12/1 -> Adder5/2(In2)  "<signal1>"
  Bus Selector10/1 -> Adder5/1(In1)  "<signal1>"
  Bus Creator18/1 -> Bus Selector2/1
  Bus Creator13/1 -> Bus Selector/1
  Bus Selector11/2 -> Adder7/1(In1)  "<signal2>"
  Bus Selector13/2 -> Adder7/2(In2)  "<signal2>"
  Adder7/2(Out2) -> Bus Creator/1  "AddOut9"
  Adder7/1(Out1) -> Bus Creator/2  "AddOut8"
  Bus Creator/1 -> Bus Creator1/1
  Adder6/1(Out1) -> Bus Creator1/2  "AddOut7"
  Bus Creator1/1 -> Bus Creator2/1
  Adder5/1(Out1) -> Bus Creator2/2  "AddOut6"
  Bus Creator2/1 -> Bus Creator3/1
  Adder4/1(Out1) -> Bus Creator3/2  "AddOut5"
  Bus Creator3/1 -> Bus Creator4/1
  Adder3/1(Out1) -> Bus Creator4/2  "AddOut4"
  Adder2/1(Out1) -> Bus Creator5/2  "AddOut3"
  Bus Creator4/1 -> Bus Creator5/1
  Bus Creator5/1 -> Bus Creator6/1
  Adder1/1(Out1) -> Bus Creator6/2  "AddOut2"
  Bus Creator6/1 -> Bus Creator7/1
  Adder/1(Out1) -> Bus Creator7/2  "AddOut1"
  Bus Creator7/1 -> AdditionDisplay/1  "AddBus"
  Subtractor1/1(Out1) -> Bus Creator41/2  "SubOut1"
  Subtractor6/1(Out1) -> Bus Creator34/2  "SubOut6"
  Subtractor8/1(Out1) -> Bus Creator22/2  "SubOut8"
  Subtractor8/2(Out2) -> Bus Creator22/1  "SubOut9"
  Subtractor3/1(Out1) -> Bus Creator39/2  "SubOut3"
  Subtractor4/1(Out1) -> Bus Creator38/2  "SubOut4"
  Bus Selector20/2 -> Bus Selector21/1  "<signal2>"
  Bus Creator27/1 -> Bus Selector14/1
  Bus Selector15/1 -> Subtractor2/1(In1)  "<signal1>"
  Bus Selector27/1 -> Subtractor5/2(In2)  "<signal1>"
  Bus Selector15/2 -> Bus Selector22/1  "<signal2>"
  Bus Selector17/2 -> Subtractor8/1(In1)  "<signal2>"
  Bus Selector21/1 -> Subtractor2/2(In2)  "<signal1>"
  Bus Selector23/1 -> Subtractor4/1(In1)  "<signal1>"
  Bus Selector22/1 -> Subtractor3/1(In1)  "<signal1>"
  Bus Selector25/2 -> Bus Selector27/1  "<signal2>"
  Sub22/1 -> Bus Creator35/1
  Sub25/1 -> Bus Creator30/1
  Bus Creator30/1 -> Bus Creator33/2
  Bus Creator33/1 -> Bus Creator31/2
  Bus Selector14/2 -> Bus Selector15/1  "<signal2>"
  Bus Selector16/1 -> Subtractor6/1(In1)  "<signal1>"
  Bus Creator28/1 -> Bus Creator26/2
  Bus Creator40/1 -> Bus Creator41/1
  Bus Creator22/1 -> Bus Creator23/1
  Sub13/1 -> Bus Creator43/1
  Bus Creator32/1 -> Bus Selector20/1
  Sub18/1 -> Bus Creator27/1
  Bus Selector26/1 -> Subtractor5/1(In1)  "<signal1>"
  Bus Creator42/1 -> Bus Creator43/2
  Bus Creator25/1 -> Bus Creator28/2
  Sub28/1 -> Bus Creator32/1
  Bus Selector23/2 -> Bus Selector26/1  "<signal2>"
  Bus Selector18/2 -> Bus Selector19/1  "<signal2>"
  Sub23/1 -> Bus Creator36/1
  Bus Selector27/2 -> Bus Selector18/1  "<signal2>"
  Subtractor2/1(Out1) -> Bus Creator40/2  "SubOut2"
  Bus Creator39/1 -> Bus Creator40/1
  Bus Selector26/2 -> Bus Selector16/1  "<signal2>"
  Bus Selector14/1 -> Subtractor1/1(In1)  "<signal1>"
  Bus Creator29/1 -> Bus Creator30/2
  Bus Selector20/1 -> Subtractor1/2(In2)  "<signal1>"
  Bus Selector16/2 -> Bus Selector17/1  "<signal2>"
  Sub11/1 -> Bus Creator42/2
  Bus Creator23/1 -> Bus Creator34/1
  Sub12/1 -> Bus Creator42/1
  Bus Selector24/1 -> Subtractor3/2(In2)  "<signal1>"
  Sub24/1 -> Bus Creator29/1
  Bus Creator26/1 -> Bus Creator27/2
  Sub26/1 -> Bus Creator33/1
  Bus Selector19/1 -> Subtractor7/2(In2)  "<signal1>"
  Sub14/1 -> Bus Creator24/1
  Bus Creator41/1 -> Display1/1  "SubBus"
  Sub15/1 -> Bus Creator25/1
  Subtractor4/2(Out2) -> Subtractor5/3(In3)
  Bus Creator31/1 -> Bus Creator32/2
  Sub21/1 -> Bus Creator35/2
  Bus Selector22/2 -> Bus Selector23/1  "<signal2>"
  Bus Selector24/2 -> Bus Selector25/1  "<signal2>"
  Subtractor5/1(Out1) -> Bus Creator37/2  "SubOut5"
  Bus Creator43/1 -> Bus Creator24/2
  Bus Creator37/1 -> Bus Creator38/1
  Bus Selector21/2 -> Bus Selector24/1  "<signal2>"
  Bus Creator38/1 -> Bus Creator39/1
  Sub27/1 -> Bus Creator31/1
  Sub17/1 -> Bus Creator26/1
  Bus Creator35/1 -> Bus Creator36/2
  Bus Creator24/1 -> Bus Creator25/2
  Sub16/1 -> Bus Creator28/1
  Bus Creator36/1 -> Bus Creator29/2
  Bus Creator34/1 -> Bus Creator37/1
  Bus Selector17/1 -> Subtractor7/1(In1)  "<signal1>"
  Subtractor1/2(Out2) -> Subtractor2/3(In3)
  Subtractor2/2(Out2) -> Subtractor3/3(In3)
  Subtractor3/2(Out2) -> Subtractor4/3(In3)
  Bus Selector25/1 -> Subtractor4/2(In2)  "<signal1>"
  Bus Selector18/1 -> Subtractor6/2(In2)  "<signal1>"
  Subtractor6/2(Out2) -> Subtractor7/3(In3)
  Subtractor7/2(Out2) -> Subtractor8/3(In3)
  Subtractor7/1(Out1) -> Bus Creator23/2  "SubOut7"
  Bus Selector19/2 -> Subtractor8/2(In2)  "<signal2>"
  Subtractor5/2(Out2) -> Subtractor6/3(In3)
  Adder10/2(Carry) -> Adder11/3(In3)
  Adder9/2(Carry) -> Adder10/3(In3)
  Adder8/2(Carry) -> Adder9/3(In3)
  Mult24/1 -> AND8/2, AND6/2, AND4/2, AND/2
  Mult23/1 -> AND9/2, AND7/2, AND5/2, AND3/2
  Adder11/2(Carry) -> Adder13/1(In1)
  AND13/1 -> Adder13/2(In2)
  AND10/1 -> Adder14/2(In2)
  Adder14/2(Carry) -> Adder15/3(In3)
  Adder9/1(Out) -> Adder14/1(In1)
  AND12/1 -> Adder12/2(In2)
  Adder11/1(Out) -> Adder12/1(In1)
  Adder10/1(Out) -> Adder15/1(In1)
  AND11/1 -> Adder15/2(In2)
  Adder15/2(Carry) -> Adder12/3(In3)
  Mult22/1 -> AND13/2, AND12/2, AND11/2, AND10/2
  Adder12/2(Carry) -> Adder13/3(In3)
  AND3/1 -> Adder8/1(In1)
  AND4/1 -> Adder8/2(In2)
  AND5/1 -> Adder9/1(In1)
  AND6/1 -> Adder9/2(In2)
  AND8/1 -> Adder10/2(In2)
  AND9/1 -> Adder11/1(In1)
  AND/1 -> Bus Creator44/2  "MultOut8"
  Adder8/1(Out) -> Bus Creator44/1  "MultOut7"
  Adder13/1(Out) -> Adder16/1(In1)
  Adder15/1(Out) -> Adder18/1(In1)
  Mult13/1 -> AND4/1, AND5/1, AND15/1, AND11/1
  Adder12/1(Out) -> Adder19/1(In1)
  Mult11/1 -> AND8/1, AND9/1, AND13/1, AND17/1
  Mult12/1 -> AND6/1, AND7/1, AND16/1, AND12/1
  Adder16/2(Carry) -> Adder17/3(In3)
  AND14/1 -> Adder18/2(In2)
  Adder18/2(Carry) -> Adder19/3(In3)
  AND17/1 -> Adder17/2(In2)
  Mult21/1 -> AND17/2, AND16/2, AND15/2, AND14/2
  AND16/1 -> Adder16/2(In2)
  Adder13/2(Carry) -> Adder17/1(In1)
  AND15/1 -> Adder19/2(In2)
  Mult14/1 -> AND/1, AND3/1, AND14/1, AND10/1
  Adder19/2(Carry) -> Adder16/3(In3)
  Adder14/1(Out) -> Bus Creator45/1  "MultOut6"
  Adder18/1(Out) -> Bus Creator46/1  "MultOut5"
  Adder19/1(Out) -> Bus Creator47/1  "MultOut4"
  Adder16/1(Out) -> Bus Creator48/1  "MultOut3"
  Adder17/1(Out) -> Bus Creator49/1  "MultOut2"
  Adder17/2(Carry) -> Bus Creator50/1  "MultOut1"
  AND7/1 -> Adder10/1(In1)
  Bus Creator44/1 -> Bus Creator45/2
  Bus Creator45/1 -> Bus Creator46/2
  Bus Creator46/1 -> Bus Creator47/2
  Bus Creator47/1 -> Bus Creator48/2
  Bus Creator48/1 -> Bus Creator49/2
  Bus Creator49/1 -> Bus Creator50/2
  Bus Creator50/1 -> Display/1  "MultBus"

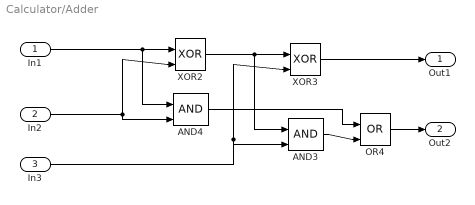
== system Calculator/Adder ==
  In1 : Inport
  In2 : Inport  Port=2
  In3 : Inport  Port=3
  AND3 : Logic  IconShape=distinctive  AllPortsSameDT=off  OutDataTypeStr=boolean
  AND4 : Logic  IconShape=distinctive  AllPortsSameDT=off  OutDataTypeStr=boolean
  OR4 : Logic  Operator=OR  IconShape=distinctive  AllPortsSameDT=off  OutDataTypeStr=boolean
  XOR2 : Logic  Operator=XOR  IconShape=distinctive  AllPortsSameDT=off  OutDataTypeStr=boolean
  XOR3 : Logic  Operator=XOR  IconShape=distinctive  AllPortsSameDT=off  OutDataTypeStr=boolean
  Out1 : Outport
  Out2 : Outport  Port=2
  wires:
  In2/1 -> AND4/2, XOR2/2
  AND3/1 -> OR4/2
  In3/1 -> XOR3/2, AND3/2
  In1/1 -> AND4/1, XOR2/1
  XOR3/1 -> Out1/1
  OR4/1 -> Out2/1
  AND4/1 -> OR4/1
  XOR2/1 -> AND3/1, XOR3/1

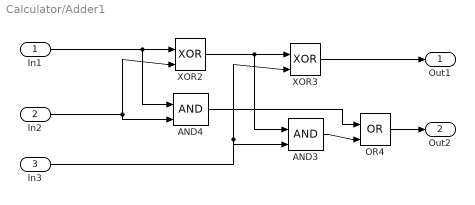
== system Calculator/Adder1 ==
  In1 : Inport
  In2 : Inport  Port=2
  In3 : Inport  Port=3
  AND3 : Logic  IconShape=distinctive  AllPortsSameDT=off  OutDataTypeStr=boolean
  AND4 : Logic  IconShape=distinctive  AllPortsSameDT=off  OutDataTypeStr=boolean
  OR4 : Logic  Operator=OR  IconShape=distinctive  AllPortsSameDT=off  OutDataTypeStr=boolean
  XOR2 : Logic  Operator=XOR  IconShape=distinctive  AllPortsSameDT=off  OutDataTypeStr=boolean
  XOR3 : Logic  Operator=XOR  IconShape=distinctive  AllPortsSameDT=off  OutDataTypeStr=boolean
  Out1 : Outport
  Out2 : Outport  Port=2
  wires:
  In2/1 -> AND4/2, XOR2/2
  AND3/1 -> OR4/2
  In3/1 -> XOR3/2, AND3/2
  In1/1 -> AND4/1, XOR2/1
  XOR3/1 -> Out1/1
  OR4/1 -> Out2/1
  AND4/1 -> OR4/1
  XOR2/1 -> AND3/1, XOR3/1

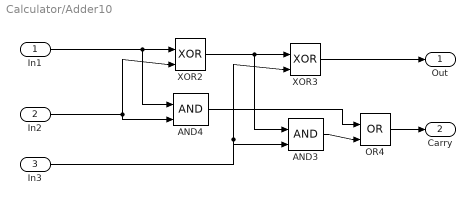
== system Calculator/Adder10 ==
  In1 : Inport
  In2 : Inport  Port=2
  In3 : Inport  Port=3
  AND3 : Logic  IconShape=distinctive  AllPortsSameDT=off  OutDataTypeStr=boolean
  AND4 : Logic  IconShape=distinctive  AllPortsSameDT=off  OutDataTypeStr=boolean
  OR4 : Logic  Operator=OR  IconShape=distinctive  AllPortsSameDT=off  OutDataTypeStr=boolean
  XOR2 : Logic  Operator=XOR  IconShape=distinctive  AllPortsSameDT=off  OutDataTypeStr=boolean
  XOR3 : Logic  Operator=XOR  IconShape=distinctive  AllPortsSameDT=off  OutDataTypeStr=boolean
  Out : Outport
  Carry : Outport  Port=2
  wires:
  In2/1 -> AND4/2, XOR2/2
  AND3/1 -> OR4/2
  In3/1 -> XOR3/2, AND3/2
  In1/1 -> AND4/1, XOR2/1
  XOR3/1 -> Out/1
  OR4/1 -> Carry/1
  AND4/1 -> OR4/1
  XOR2/1 -> AND3/1, XOR3/1

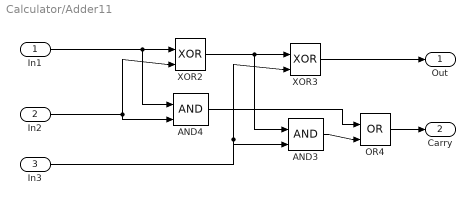
== system Calculator/Adder11 ==
  In1 : Inport
  In2 : Inport  Port=2
  In3 : Inport  Port=3
  AND3 : Logic  IconShape=distinctive  AllPortsSameDT=off  OutDataTypeStr=boolean
  AND4 : Logic  IconShape=distinctive  AllPortsSameDT=off  OutDataTypeStr=boolean
  OR4 : Logic  Operator=OR  IconShape=distinctive  AllPortsSameDT=off  OutDataTypeStr=boolean
  XOR2 : Logic  Operator=XOR  IconShape=distinctive  AllPortsSameDT=off  OutDataTypeStr=boolean
  XOR3 : Logic  Operator=XOR  IconShape=distinctive  AllPortsSameDT=off  OutDataTypeStr=boolean
  Out : Outport
  Carry : Outport  Port=2
  wires:
  In2/1 -> AND4/2, XOR2/2
  AND3/1 -> OR4/2
  In3/1 -> XOR3/2, AND3/2
  In1/1 -> AND4/1, XOR2/1
  XOR3/1 -> Out/1
  OR4/1 -> Carry/1
  AND4/1 -> OR4/1
  XOR2/1 -> AND3/1, XOR3/1

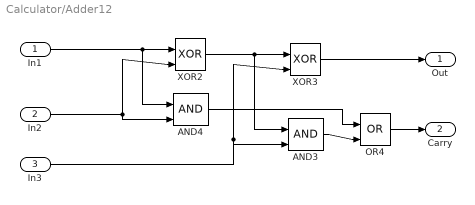
== system Calculator/Adder12 ==
  In1 : Inport
  In2 : Inport  Port=2
  In3 : Inport  Port=3
  AND3 : Logic  IconShape=distinctive  AllPortsSameDT=off  OutDataTypeStr=boolean
  AND4 : Logic  IconShape=distinctive  AllPortsSameDT=off  OutDataTypeStr=boolean
  OR4 : Logic  Operator=OR  IconShape=distinctive  AllPortsSameDT=off  OutDataTypeStr=boolean
  XOR2 : Logic  Operator=XOR  IconShape=distinctive  AllPortsSameDT=off  OutDataTypeStr=boolean
  XOR3 : Logic  Operator=XOR  IconShape=distinctive  AllPortsSameDT=off  OutDataTypeStr=boolean
  Out : Outport
  Carry : Outport  Port=2
  wires:
  In2/1 -> AND4/2, XOR2/2
  AND3/1 -> OR4/2
  In3/1 -> XOR3/2, AND3/2
  In1/1 -> AND4/1, XOR2/1
  XOR3/1 -> Out/1
  OR4/1 -> Carry/1
  AND4/1 -> OR4/1
  XOR2/1 -> AND3/1, XOR3/1

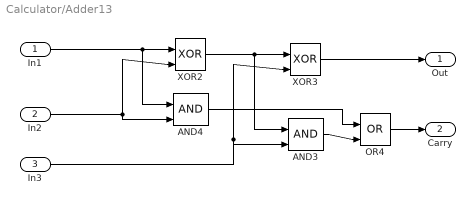
== system Calculator/Adder13 ==
  In1 : Inport
  In2 : Inport  Port=2
  In3 : Inport  Port=3
  AND3 : Logic  IconShape=distinctive  AllPortsSameDT=off  OutDataTypeStr=boolean
  AND4 : Logic  IconShape=distinctive  AllPortsSameDT=off  OutDataTypeStr=boolean
  OR4 : Logic  Operator=OR  IconShape=distinctive  AllPortsSameDT=off  OutDataTypeStr=boolean
  XOR2 : Logic  Operator=XOR  IconShape=distinctive  AllPortsSameDT=off  OutDataTypeStr=boolean
  XOR3 : Logic  Operator=XOR  IconShape=distinctive  AllPortsSameDT=off  OutDataTypeStr=boolean
  Out : Outport
  Carry : Outport  Port=2
  wires:
  In2/1 -> AND4/2, XOR2/2
  AND3/1 -> OR4/2
  In3/1 -> XOR3/2, AND3/2
  In1/1 -> AND4/1, XOR2/1
  XOR3/1 -> Out/1
  OR4/1 -> Carry/1
  AND4/1 -> OR4/1
  XOR2/1 -> AND3/1, XOR3/1

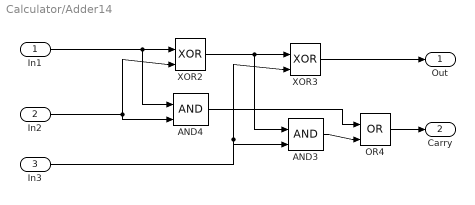
== system Calculator/Adder14 ==
  In1 : Inport
  In2 : Inport  Port=2
  In3 : Inport  Port=3
  AND3 : Logic  IconShape=distinctive  AllPortsSameDT=off  OutDataTypeStr=boolean
  AND4 : Logic  IconShape=distinctive  AllPortsSameDT=off  OutDataTypeStr=boolean
  OR4 : Logic  Operator=OR  IconShape=distinctive  AllPortsSameDT=off  OutDataTypeStr=boolean
  XOR2 : Logic  Operator=XOR  IconShape=distinctive  AllPortsSameDT=off  OutDataTypeStr=boolean
  XOR3 : Logic  Operator=XOR  IconShape=distinctive  AllPortsSameDT=off  OutDataTypeStr=boolean
  Out : Outport
  Carry : Outport  Port=2
  wires:
  In2/1 -> AND4/2, XOR2/2
  AND3/1 -> OR4/2
  In3/1 -> XOR3/2, AND3/2
  In1/1 -> AND4/1, XOR2/1
  XOR3/1 -> Out/1
  OR4/1 -> Carry/1
  AND4/1 -> OR4/1
  XOR2/1 -> AND3/1, XOR3/1

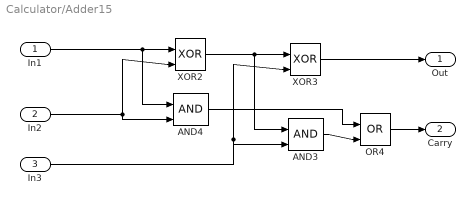
== system Calculator/Adder15 ==
  In1 : Inport
  In2 : Inport  Port=2
  In3 : Inport  Port=3
  AND3 : Logic  IconShape=distinctive  AllPortsSameDT=off  OutDataTypeStr=boolean
  AND4 : Logic  IconShape=distinctive  AllPortsSameDT=off  OutDataTypeStr=boolean
  OR4 : Logic  Operator=OR  IconShape=distinctive  AllPortsSameDT=off  OutDataTypeStr=boolean
  XOR2 : Logic  Operator=XOR  IconShape=distinctive  AllPortsSameDT=off  OutDataTypeStr=boolean
  XOR3 : Logic  Operator=XOR  IconShape=distinctive  AllPortsSameDT=off  OutDataTypeStr=boolean
  Out : Outport
  Carry : Outport  Port=2
  wires:
  In2/1 -> AND4/2, XOR2/2
  AND3/1 -> OR4/2
  In3/1 -> XOR3/2, AND3/2
  In1/1 -> AND4/1, XOR2/1
  XOR3/1 -> Out/1
  OR4/1 -> Carry/1
  AND4/1 -> OR4/1
  XOR2/1 -> AND3/1, XOR3/1

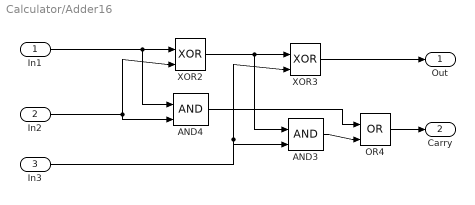
== system Calculator/Adder16 ==
  In1 : Inport
  In2 : Inport  Port=2
  In3 : Inport  Port=3
  AND3 : Logic  IconShape=distinctive  AllPortsSameDT=off  OutDataTypeStr=boolean
  AND4 : Logic  IconShape=distinctive  AllPortsSameDT=off  OutDataTypeStr=boolean
  OR4 : Logic  Operator=OR  IconShape=distinctive  AllPortsSameDT=off  OutDataTypeStr=boolean
  XOR2 : Logic  Operator=XOR  IconShape=distinctive  AllPortsSameDT=off  OutDataTypeStr=boolean
  XOR3 : Logic  Operator=XOR  IconShape=distinctive  AllPortsSameDT=off  OutDataTypeStr=boolean
  Out : Outport
  Carry : Outport  Port=2
  wires:
  In2/1 -> AND4/2, XOR2/2
  AND3/1 -> OR4/2
  In3/1 -> XOR3/2, AND3/2
  In1/1 -> AND4/1, XOR2/1
  XOR3/1 -> Out/1
  OR4/1 -> Carry/1
  AND4/1 -> OR4/1
  XOR2/1 -> AND3/1, XOR3/1

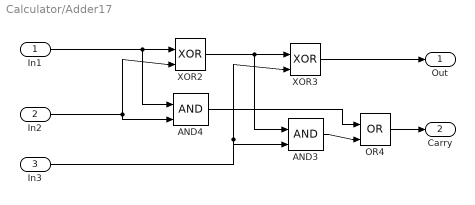
== system Calculator/Adder17 ==
  In1 : Inport
  In2 : Inport  Port=2
  In3 : Inport  Port=3
  AND3 : Logic  IconShape=distinctive  AllPortsSameDT=off  OutDataTypeStr=boolean
  AND4 : Logic  IconShape=distinctive  AllPortsSameDT=off  OutDataTypeStr=boolean
  OR4 : Logic  Operator=OR  IconShape=distinctive  AllPortsSameDT=off  OutDataTypeStr=boolean
  XOR2 : Logic  Operator=XOR  IconShape=distinctive  AllPortsSameDT=off  OutDataTypeStr=boolean
  XOR3 : Logic  Operator=XOR  IconShape=distinctive  AllPortsSameDT=off  OutDataTypeStr=boolean
  Out : Outport
  Carry : Outport  Port=2
  wires:
  In2/1 -> AND4/2, XOR2/2
  AND3/1 -> OR4/2
  In3/1 -> XOR3/2, AND3/2
  In1/1 -> AND4/1, XOR2/1
  XOR3/1 -> Out/1
  OR4/1 -> Carry/1
  AND4/1 -> OR4/1
  XOR2/1 -> AND3/1, XOR3/1

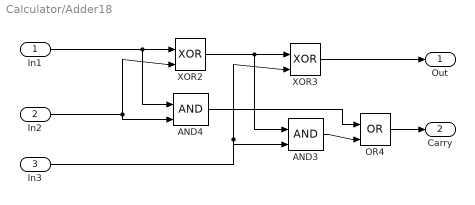
== system Calculator/Adder18 ==
  In1 : Inport
  In2 : Inport  Port=2
  In3 : Inport  Port=3
  AND3 : Logic  IconShape=distinctive  AllPortsSameDT=off  OutDataTypeStr=boolean
  AND4 : Logic  IconShape=distinctive  AllPortsSameDT=off  OutDataTypeStr=boolean
  OR4 : Logic  Operator=OR  IconShape=distinctive  AllPortsSameDT=off  OutDataTypeStr=boolean
  XOR2 : Logic  Operator=XOR  IconShape=distinctive  AllPortsSameDT=off  OutDataTypeStr=boolean
  XOR3 : Logic  Operator=XOR  IconShape=distinctive  AllPortsSameDT=off  OutDataTypeStr=boolean
  Out : Outport
  Carry : Outport  Port=2
  wires:
  In2/1 -> AND4/2, XOR2/2
  AND3/1 -> OR4/2
  In3/1 -> XOR3/2, AND3/2
  In1/1 -> AND4/1, XOR2/1
  XOR3/1 -> Out/1
  OR4/1 -> Carry/1
  AND4/1 -> OR4/1
  XOR2/1 -> AND3/1, XOR3/1

== system Calculator/Adder19 ==
  In1 : Inport
  In2 : Inport  Port=2
  In3 : Inport  Port=3
  AND3 : Logic  IconShape=distinctive  AllPortsSameDT=off  OutDataTypeStr=boolean
  AND4 : Logic  IconShape=distinctive  AllPortsSameDT=off  OutDataTypeStr=boolean
  OR4 : Logic  Operator=OR  IconShape=distinctive  AllPortsSameDT=off  OutDataTypeStr=boolean
  XOR2 : Logic  Operator=XOR  IconShape=distinctive  AllPortsSameDT=off  OutDataTypeStr=boolean
  XOR3 : Logic  Operator=XOR  IconShape=distinctive  AllPortsSameDT=off  OutDataTypeStr=boolean
  Out : Outport
  Carry : Outport  Port=2
  wires:
  In2/1 -> AND4/2, XOR2/2
  AND3/1 -> OR4/2
  In3/1 -> XOR3/2, AND3/2
  In1/1 -> AND4/1, XOR2/1
  XOR3/1 -> Out/1
  OR4/1 -> Carry/1
  AND4/1 -> OR4/1
  XOR2/1 -> AND3/1, XOR3/1

== system Calculator/Adder2 ==
  In1 : Inport
  In2 : Inport  Port=2
  In3 : Inport  Port=3
  AND3 : Logic  IconShape=distinctive  AllPortsSameDT=off  OutDataTypeStr=boolean
  AND4 : Logic  IconShape=distinctive  AllPortsSameDT=off  OutDataTypeStr=boolean
  OR4 : Logic  Operator=OR  IconShape=distinctive  AllPortsSameDT=off  OutDataTypeStr=boolean
  XOR2 : Logic  Operator=XOR  IconShape=distinctive  AllPortsSameDT=off  OutDataTypeStr=boolean
  XOR3 : Logic  Operator=XOR  IconShape=distinctive  AllPortsSameDT=off  OutDataTypeStr=boolean
  Out1 : Outport
  Out2 : Outport  Port=2
  wires:
  In2/1 -> AND4/2, XOR2/2
  AND3/1 -> OR4/2
  In3/1 -> XOR3/2, AND3/2
  In1/1 -> AND4/1, XOR2/1
  XOR3/1 -> Out1/1
  OR4/1 -> Out2/1
  AND4/1 -> OR4/1
  XOR2/1 -> AND3/1, XOR3/1

== system Calculator/Adder3 ==
  In1 : Inport
  In2 : Inport  Port=2
  In3 : Inport  Port=3
  AND3 : Logic  IconShape=distinctive  AllPortsSameDT=off  OutDataTypeStr=boolean
  AND4 : Logic  IconShape=distinctive  AllPortsSameDT=off  OutDataTypeStr=boolean
  OR4 : Logic  Operator=OR  IconShape=distinctive  AllPortsSameDT=off  OutDataTypeStr=boolean
  XOR2 : Logic  Operator=XOR  IconShape=distinctive  AllPortsSameDT=off  OutDataTypeStr=boolean
  XOR3 : Logic  Operator=XOR  IconShape=distinctive  AllPortsSameDT=off  OutDataTypeStr=boolean
  Out1 : Outport
  Out2 : Outport  Port=2
  wires:
  In2/1 -> AND4/2, XOR2/2
  AND3/1 -> OR4/2
  In3/1 -> XOR3/2, AND3/2
  In1/1 -> AND4/1, XOR2/1
  XOR3/1 -> Out1/1
  OR4/1 -> Out2/1
  AND4/1 -> OR4/1
  XOR2/1 -> AND3/1, XOR3/1

== system Calculator/Adder4 ==
  In1 : Inport
  In2 : Inport  Port=2
  In3 : Inport  Port=3
  AND3 : Logic  IconShape=distinctive  AllPortsSameDT=off  OutDataTypeStr=boolean
  AND4 : Logic  IconShape=distinctive  AllPortsSameDT=off  OutDataTypeStr=boolean
  OR4 : Logic  Operator=OR  IconShape=distinctive  AllPortsSameDT=off  OutDataTypeStr=boolean
  XOR2 : Logic  Operator=XOR  IconShape=distinctive  AllPortsSameDT=off  OutDataTypeStr=boolean
  XOR3 : Logic  Operator=XOR  IconShape=distinctive  AllPortsSameDT=off  OutDataTypeStr=boolean
  Out1 : Outport
  Out2 : Outport  Port=2
  wires:
  In2/1 -> AND4/2, XOR2/2
  AND3/1 -> OR4/2
  In3/1 -> XOR3/2, AND3/2
  In1/1 -> AND4/1, XOR2/1
  XOR3/1 -> Out1/1
  OR4/1 -> Out2/1
  AND4/1 -> OR4/1
  XOR2/1 -> AND3/1, XOR3/1

== system Calculator/Adder5 ==
  In1 : Inport
  In2 : Inport  Port=2
  In3 : Inport  Port=3
  AND3 : Logic  IconShape=distinctive  AllPortsSameDT=off  OutDataTypeStr=boolean
  AND4 : Logic  IconShape=distinctive  AllPortsSameDT=off  OutDataTypeStr=boolean
  OR4 : Logic  Operator=OR  IconShape=distinctive  AllPortsSameDT=off  OutDataTypeStr=boolean
  XOR2 : Logic  Operator=XOR  IconShape=distinctive  AllPortsSameDT=off  OutDataTypeStr=boolean
  XOR3 : Logic  Operator=XOR  IconShape=distinctive  AllPortsSameDT=off  OutDataTypeStr=boolean
  Out1 : Outport
  Out2 : Outport  Port=2
  wires:
  In2/1 -> AND4/2, XOR2/2
  AND3/1 -> OR4/2
  In3/1 -> XOR3/2, AND3/2
  In1/1 -> AND4/1, XOR2/1
  XOR3/1 -> Out1/1
  OR4/1 -> Out2/1
  AND4/1 -> OR4/1
  XOR2/1 -> AND3/1, XOR3/1

== system Calculator/Adder6 ==
  In1 : Inport
  In2 : Inport  Port=2
  In3 : Inport  Port=3
  AND3 : Logic  IconShape=distinctive  AllPortsSameDT=off  OutDataTypeStr=boolean
  AND4 : Logic  IconShape=distinctive  AllPortsSameDT=off  OutDataTypeStr=boolean
  OR4 : Logic  Operator=OR  IconShape=distinctive  AllPortsSameDT=off  OutDataTypeStr=boolean
  XOR2 : Logic  Operator=XOR  IconShape=distinctive  AllPortsSameDT=off  OutDataTypeStr=boolean
  XOR3 : Logic  Operator=XOR  IconShape=distinctive  AllPortsSameDT=off  OutDataTypeStr=boolean
  Out1 : Outport
  Out2 : Outport  Port=2
  wires:
  In2/1 -> AND4/2, XOR2/2
  AND3/1 -> OR4/2
  In3/1 -> XOR3/2, AND3/2
  In1/1 -> AND4/1, XOR2/1
  XOR3/1 -> Out1/1
  OR4/1 -> Out2/1
  AND4/1 -> OR4/1
  XOR2/1 -> AND3/1, XOR3/1
